simulink model "FIR_filter"  (R2020a)
settings: Solver=VariableStepAuto  StartTime=0.0  StopTime=10.0  RelTol=1e-3
settings Model: Creator=DELL  LastModifiedBy=DELL

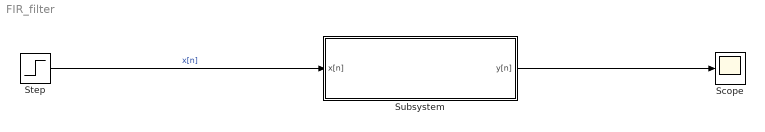
== system FIR_filter ==
  Scope : Scope
  Step : Step  SampleTime=0
  Subsystem : Subsystem
  wires:
  Step/1 -> Subsystem/1(x[n])  "x[n]"
  Subsystem/1(y[n]) -> Scope/1

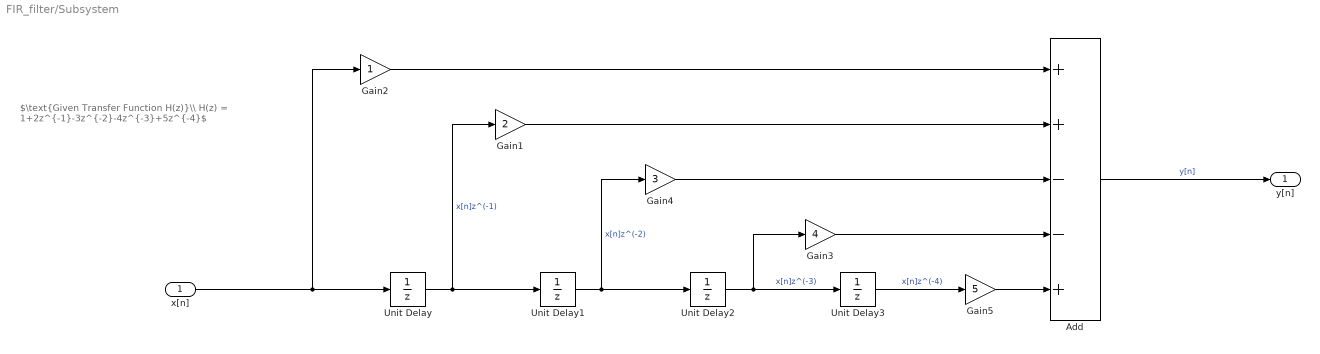
== system FIR_filter/Subsystem ==
  note: $\text{Given Transfer Function H(z)}\\ H(z) = 1+2z^{-1}-3z^{-2}-4z^{-3}+5z^{-4}$
  x[n] : Inport
  Add : Sum  Inputs=++--+
  Gain1 : Gain  Gain=2
  Gain2 : Gain
  Gain3 : Gain  Gain=4
  Gain4 : Gain  Gain=3
  Gain5 : Gain  Gain=5
  Unit Delay{,1..3} (4 alike) : UnitDelay  SampleTime=-1  HasFrameUpgradeWarning=on
  y[n] : Outport
  wires:
  Gain3/1 -> Add/4
  x[n]/1 -> Unit Delay/1, Gain2/1
  Gain2/1 -> Add/1
  Unit Delay1/1 -> Gain4/1, Unit Delay2/1  "x[n]z^(-2)"
  Gain5/1 -> Add/5
  Unit Delay2/1 -> Gain3/1, Unit Delay3/1  "x[n]z^(-3)"
  Gain4/1 -> Add/3
  Unit Delay/1 -> Gain1/1, Unit Delay1/1  "x[n]z^(-1)"
  Gain1/1 -> Add/2
  Unit Delay3/1 -> Gain5/1  "x[n]z^(-4)"
  Add/1 -> y[n]/1  "y[n]"
